simulink library "BlockLibrary"  (R2022b)
settings: Solver=VariableStepAuto  StartTime=0.0  StopTime=10.0  RelTol=1e-3
undefined symbols (not defined in the file or in its folder): DiscIntNeverNeededParam
libraries: simulink x1
settings Model: Creator=Kevin  LastModifiedBy=Kevin

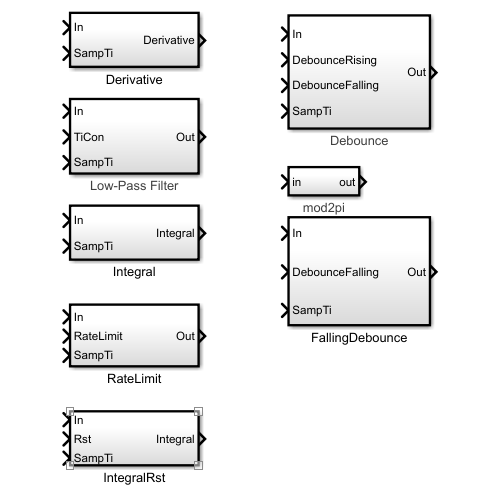
[thumbnail: Simulink's stored preview of the top-level diagram]
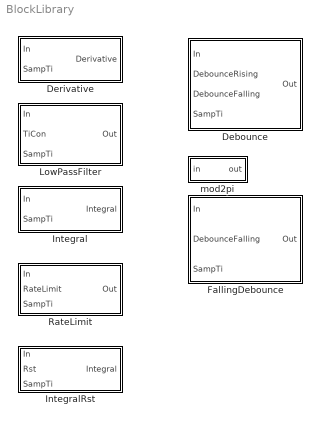
== system BlockLibrary ==
  Debounce : Subsystem  Description=Debounce  TreatAsAtomicUnit=on
      settings: AttributesFormatString=%<Description>
  Derivative : Subsystem  TreatAsAtomicUnit=on
  FallingDebounce : Subsystem  TreatAsAtomicUnit=on
  Integral : Subsystem  TreatAsAtomicUnit=on
  IntegralRst : Subsystem  TreatAsAtomicUnit=on
  LowPassFilter : Subsystem  Description=Low-Pass Filter  TreatAsAtomicUnit=on
      settings: AttributesFormatString=%<Description>
  RateLimit : Subsystem  TreatAsAtomicUnit=on
  mod2pi : Subsystem  Description=mod2pi  TreatAsAtomicUnit=on
      settings: AttributesFormatString=%<Description>

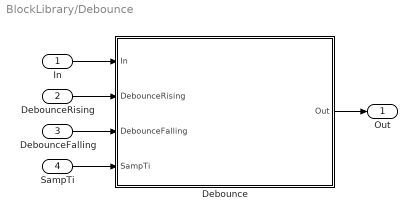
== system BlockLibrary/Debounce ==
  In : Inport
  DebounceRising : Inport  Port=2
  DebounceFalling : Inport  Port=3
  SampTi : Inport  Port=4
  Debounce : Stateflow chart  TreatAsAtomicUnit=on
      settings: PortSchema="{\"entries\":[{\"content\":{\"sides\":[{\"content\":{\"connectorIds\":[\"In4\",\"In2\",\"In3\",\"In1\"]},\"type\":\"ConnectorPlacement.EquallySpacedRectSide\",\"uuid\":\"aecadd78-b999-472c-9e3b-112da4c892dc\"},{\"content\":{\"connectorIds\":[\"Out1\"],\"side\":\"RIGHT\"},\"type\":\"ConnectorPlacement.EquallySpacedRectSide\",\"uuid\":\"38577757-9ea5-4cd3-a261-520b3734182a\"},{\"content\":{\"connectorIds\":[],\"side\":\"TOP\"},\"type\":\"ConnectorPlacement.EquallySpacedRectSide\",\"uuid\":\"bee6da78-0990-44a0-aa9d-c8a80681ba83\"}]},\"type\":\"ConnectorPlacement.EquallySpacedConnector\",\"uuid\":\"415f8257-0027-45f8-948a-946df9b54cde\"}],\"packageUris\":[\"http://schema.mathworks.com/mf0/Connector/R2020b\"],\"version\":\"1.0\"}"
  Out : Outport
  wires:
  In/1 -> Debounce/4(In)
  DebounceRising/1 -> Debounce/2(DebounceRising)
  DebounceFalling/1 -> Debounce/3(DebounceFalling)
  SampTi/1 -> Debounce/1(SampTi)
  Debounce/1(Out) -> Out/1

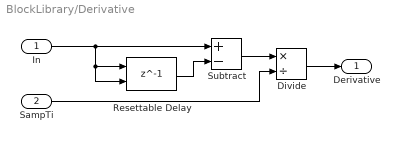
== system BlockLibrary/Derivative ==
  In : Inport
  SampTi : Inport  Port=2
  Divide : Product  Inputs=*/
  Resettable Delay : Delay  DelayLength=1  InitialConditionSource=Input port
      settings: InputPortMap=u0,p4
  Subtract : Sum  Inputs=+-
  Derivative : Outport
  wires:
  In/1 -> Subtract/1, Resettable Delay/2, Resettable Delay/1
  Resettable Delay/1 -> Subtract/2
  Subtract/1 -> Divide/1
  Divide/1 -> Derivative/1
  SampTi/1 -> Divide/2

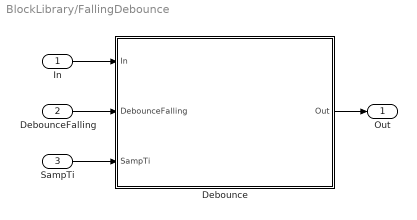
== system BlockLibrary/FallingDebounce ==
  In : Inport
  DebounceFalling : Inport  Port=2
  SampTi : Inport  Port=3
  Debounce : Stateflow chart  TreatAsAtomicUnit=on
      settings: PortSchema="{\"entries\":[{\"content\":{\"sides\":[{\"content\":{\"connectorIds\":[\"In3\",\"In2\",\"In1\"]},\"type\":\"ConnectorPlacement.EquallySpacedRectSide\",\"uuid\":\"aecadd78-b999-472c-9e3b-112da4c892dc\"},{\"content\":{\"connectorIds\":[\"Out1\"],\"side\":\"RIGHT\"},\"type\":\"ConnectorPlacement.EquallySpacedRectSide\",\"uuid\":\"38577757-9ea5-4cd3-a261-520b3734182a\"},{\"content\":{\"connectorIds\":[],\"side\":\"TOP\"},\"type\":\"ConnectorPlacement.EquallySpacedRectSide\",\"uuid\":\"bee6da78-0990-44a0-aa9d-c8a80681ba83\"}]},\"type\":\"ConnectorPlacement.EquallySpacedConnector\",\"uuid\":\"415f8257-0027-45f8-948a-946df9b54cde\"}],\"packageUris\":[\"http://schema.mathworks.com/mf0/Connector/R2020b\"],\"version\":\"1.0\"}"
  Out : Outport
  wires:
  Debounce/1(Out) -> Out/1
  SampTi/1 -> Debounce/1(SampTi)
  DebounceFalling/1 -> Debounce/2(DebounceFalling)
  In/1 -> Debounce/3(In)

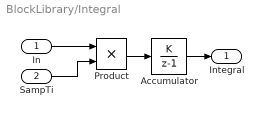
== system BlockLibrary/Integral ==
  In : Inport
  SampTi : Inport  Port=2
  Accumulator : DiscreteIntegrator  IntegratorMethod=Accumulation: Forward Euler  SampleTime=-1  ICPrevOutput=DiscIntNeverNeededParam  ICPrevScaledInput=DiscIntNeverNeededParam
  Product : Product
  Integral : Outport
  wires:
  SampTi/1 -> Product/2
  Accumulator/1 -> Integral/1
  In/1 -> Product/1
  Product/1 -> Accumulator/1

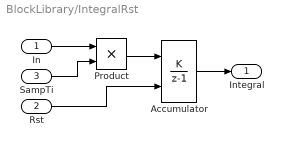
== system BlockLibrary/IntegralRst ==
  In : Inport
  Rst : Inport  Port=2
  SampTi : Inport  Port=3
  Accumulator : DiscreteIntegrator  IntegratorMethod=Accumulation: Forward Euler  ExternalReset=level  SampleTime=-1  ICPrevOutput=DiscIntNeverNeededParam  ICPrevScaledInput=DiscIntNeverNeededParam
  Product : Product
  Integral : Outport
  wires:
  Product/1 -> Accumulator/1
  In/1 -> Product/1
  Accumulator/1 -> Integral/1
  SampTi/1 -> Product/2
  Rst/1 -> Accumulator/2

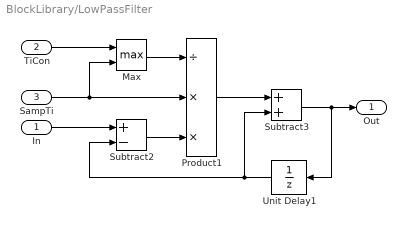
== system BlockLibrary/LowPassFilter ==
  In : Inport
  TiCon : Inport  Port=2
  SampTi : Inport  Port=3
  Max : MinMax  Function=max  Inputs=2
  Product1 : Product  Inputs=/**
  Subtract2 : Sum  Inputs=+-
  Subtract3 : Sum
  Unit Delay1 : UnitDelay  SampleTime=-1  HasFrameUpgradeWarning=on
  Out : Outport
  wires:
  Subtract3/1 -> Unit Delay1/1, Out/1
  Unit Delay1/1 -> Subtract2/2, Subtract3/2
  Product1/1 -> Subtract3/1
  Subtract2/1 -> Product1/3
  In/1 -> Subtract2/1
  TiCon/1 -> Max/1
  SampTi/1 -> Product1/2, Max/2
  Max/1 -> Product1/1

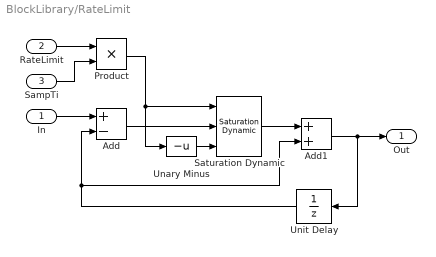
== system BlockLibrary/RateLimit ==
  In : Inport
  RateLimit : Inport  Port=2
  SampTi : Inport  Port=3
  Add : Sum  Inputs=+-
  Add1 : Sum
  Product : Product
  Saturation Dynamic : simulink/Discontinuities/Saturation Dynamic  OutMin=[]  OutMax=[]  OutDataTypeStr=Inherit: Same as second input  OutDataType=fixdt(1, 16)  OutScaling=2^-10  DoSatur=off
  Unary Minus : UnaryMinus
  Unit Delay : UnitDelay  SampleTime=-1  HasFrameUpgradeWarning=on
  Out : Outport
  wires:
  Add1/1 -> Out/1, Unit Delay/1
  SampTi/1 -> Product/2
  RateLimit/1 -> Product/1
  In/1 -> Add/1
  Unit Delay/1 -> Add/2, Add1/2
  Saturation Dynamic/1 -> Add1/1
  Add/1 -> Saturation Dynamic/2
  Unary Minus/1 -> Saturation Dynamic/3
  Product/1 -> Unary Minus/1, Saturation Dynamic/1

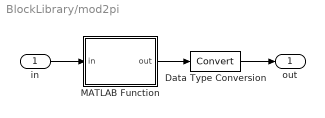
== system BlockLibrary/mod2pi ==
  in : Inport
  Data Type Conversion : DataTypeConversion  SaturateOnIntegerOverflow=off  RndMeth=Floor
  MATLAB Function : MATLAB Function  TreatAsAtomicUnit=on
  out : Outport
  wires:
  in/1 -> MATLAB Function/1(in)
  MATLAB Function/1(out) -> Data Type Conversion/1
  Data Type Conversion/1 -> out/1

== stateflow chart BlockLibrary/FallingDebounce/Debounce ==
  state INACTIVE
    Out = false;
    Tmr = 0;
  state ACTIVE_WAIT
    du:
    Out = true;
    Tmr = Tmr + SampTi;
  state ACTIVE
    Out = true;
    Tmr = 0;
  (default) -> INACTIVE
  ACTIVE_WAIT -> INACTIVE [order 2] : [Tmr >= DebounceFalling]
  INACTIVE -> (junction 19) : [In]
  ACTIVE_WAIT -> ACTIVE [order 1] : [In]
  ACTIVE -> ACTIVE_WAIT : [~In]
  (junction 19) -> ACTIVE
  data: SampTi input; DebounceFalling input; Out output; In input; Tmr local single

== matlab function BlockLibrary/mod2pi/MATLAB Function ==
  data: in input; out output
function out = fcn(in)
temp = in;
pi2 = 6.2831;
while temp > pi2
    temp = temp - pi2;
end
while temp < 0
    temp = temp + pi2;
end
out = temp;

== stateflow chart BlockLibrary/Debounce/Debounce ==
  state INACTIVE
    Out = false;
    Tmr = 0;
  state ACTIVE_WAIT
    du:
    Out = true;
    Tmr = Tmr + SampTi;
  state INACTIVE_WAIT
    Out = false;
    Tmr = Tmr + SampTi;
  state ACTIVE
    Out = true;
    Tmr = 0;
  (default) -> INACTIVE
  ACTIVE_WAIT -> INACTIVE [order 2] : [Tmr >= DebounceFalling]
  INACTIVE -> INACTIVE_WAIT : [In]
  INACTIVE_WAIT -> INACTIVE [order 1] : [~In]
  ACTIVE_WAIT -> ACTIVE [order 1] : [In]
  ACTIVE -> ACTIVE_WAIT : [~In]
  INACTIVE_WAIT -> ACTIVE [order 2] : [Tmr >= DebounceRising]
  data: SampTi input; DebounceRising input; DebounceFalling input; Out output; In input; Tmr local single
